simulink model "Model_complet"  (R2016a)
settings: Solver=VariableStepAuto  StartTime=0.0  StopTime=0.3  RelTol=1e-3
values from neighbouring files (symbols this model uses):
  Kid_ = 1*a1^2/e1    (= 5500.9287619)    [Data.m]
  Kiq_ = 1*b2^2/e2    (= 3122.67350797)    [Data.m]
  Pd_ = -1*a1/e1    (= 12.8976)    [Data.m]
  Pq_ = -1*b2/e2    (= 11.452173913)    [Data.m]
settings Model: Creator=NAD  LastModifiedBy=NAD

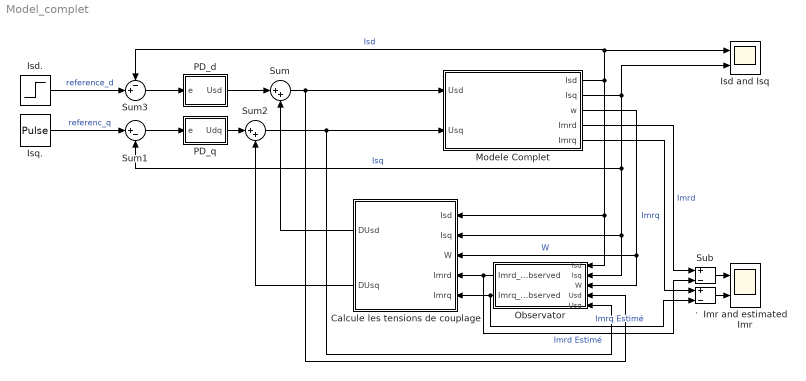
== system Model_complet ==
  . : Sum  Inputs=+-
  Calcule les tensions de couplage : MATLAB Function  TreatAsAtomicUnit=on
  Imr and estimated Imr : Scope  NumInputPorts=2
  Isd and Isq : Scope  NumInputPorts=2
  Isd. : Step  Time=0  After=10  SampleTime=0
  Isq. : DiscretePulseGenerator  PulseType=Time based  Amplitude=10  Period=0.2  PulseWidth=50
  Modele Complet : Subsystem
  Observator : Subsystem
  PD_d : Subsystem
  PD_q : Subsystem
  Sub : Sum  Inputs=+-
  Sum : Sum  Inputs=|++
  Sum1 : Sum  Inputs=|+-
  Sum2 : Sum  Inputs=|++
  Sum3 : Sum  Inputs=-+|
  wires:
  Modele Complet/1(Isd) -> Calcule les tensions de couplage/1(Isd), Observator/1(Isd), Sum3/1, Isd and Isq/1  "Isd"
  Modele Complet/3(w) -> Calcule les tensions de couplage/3(W), Observator/3(W)  "W"
  Sum3/1 -> PD_d/1(e)
  Sum1/1 -> PD_q/1(e)
  PD_d/1(Usd) -> Sum/1
  Sum/1 -> Observator/4(Usd), Modele Complet/1(Usd)
  Sum2/1 -> Observator/5(Usq), Modele Complet/2(Usq)
  PD_q/1(Udq) -> Sum2/1
  Calcule les tensions de couplage/1(DUsd) -> Sum/2
  Calcule les tensions de couplage/2(DUsq) -> Sum2/2
  Observator/1(Imrd_Observed) -> Sub/2, Calcule les tensions de couplage/4(Imrd)  "Imrd Estimé"
  Observator/2(Imrq_Observed) -> ./2, Calcule les tensions de couplage/5(Imrq)  "Imrq Estimé"
  Sub/1 -> Imr and estimated Imr/1
  Modele Complet/4(Imrd) -> Sub/1  "Imrd"
  Modele Complet/5(Imrq) -> ./1  "Imrq"
  ./1 -> Imr and estimated Imr/2
  Modele Complet/2(Isq) -> Sum1/2, Calcule les tensions de couplage/2(Isq), Observator/2(Isq), Isd and Isq/2  "Isq"
  Isq./1 -> Sum1/1  "referenc_q"
  Isd./1 -> Sum3/2  "reference_d"

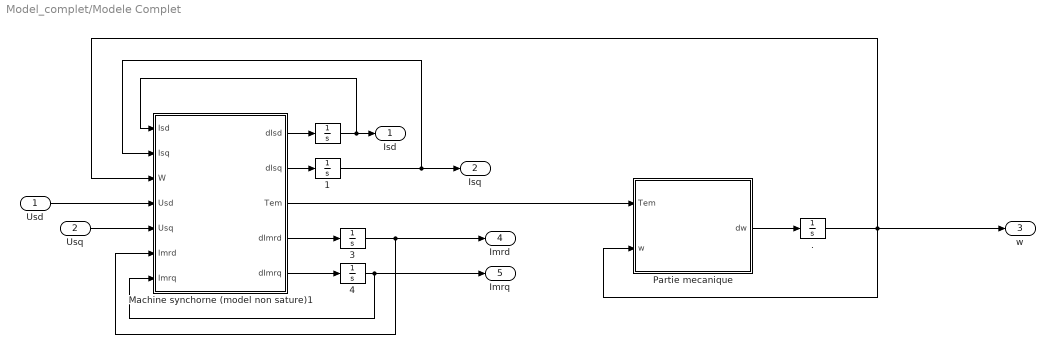
== system Model_complet/Modele Complet ==
  Usd : Inport
  Usq : Inport  Port=2
  " " : Integrator
  " ." : Integrator
  " 1" : Integrator
  " 3" : Integrator  InitialCondition=1
  " 4" : Integrator  InitialCondition=1
  Machine synchorne (model non sature)1 : MATLAB Function  TreatAsAtomicUnit=on
  Partie mecanique : MATLAB Function  TreatAsAtomicUnit=on
  Isd : Outport
  Isq : Outport  Port=2
  w : Outport  Port=3
  Imrd : Outport  Port=4
  Imrq : Outport  Port=5
  wires:
  Machine synchorne (model non sature)1/1(dIsd) -> " "/1
  " "/1 -> Isd/1, Machine synchorne (model non sature)1/1(Isd)
  " ."/1 -> w/1, Partie mecanique/2(w), Machine synchorne (model non sature)1/3(W)
  Partie mecanique/1(dw) -> " ."/1
  Machine synchorne (model non sature)1/3(Tem) -> Partie mecanique/1(Tem)
  Machine synchorne (model non sature)1/2(dIsq) -> " 1"/1
  " 1"/1 -> Machine synchorne (model non sature)1/2(Isq), Isq/1
  Usd/1 -> Machine synchorne (model non sature)1/4(Usd)
  Usq/1 -> Machine synchorne (model non sature)1/5(Usq)
  Machine synchorne (model non sature)1/4(dImrd) -> " 3"/1
  Machine synchorne (model non sature)1/5(dImrq) -> " 4"/1
  " 4"/1 -> Machine synchorne (model non sature)1/7(Imrq), Imrq/1
  " 3"/1 -> Imrd/1, Machine synchorne (model non sature)1/6(Imrd)

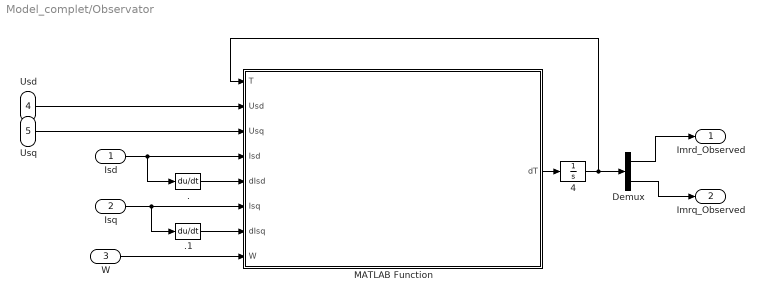
== system Model_complet/Observator ==
  Isd : Inport
  Isq : Inport  Port=2
  W : Inport  Port=3
  Usd : Inport  Port=4
  Usq : Inport  Port=5
  " 4" : Integrator  InitialCondition=0.01*[1;1]
  . : Derivative
  .1 : Derivative
  Demux : Demux  Outputs=2
  MATLAB Function : MATLAB Function  TreatAsAtomicUnit=on
  Imrd_Observed : Outport
  Imrq_Observed : Outport  Port=2
  wires:
  W/1 -> MATLAB Function/8(W)
  .1/1 -> MATLAB Function/7(dIsq)
  MATLAB Function/1(dT) -> " 4"/1
  " 4"/1 -> Demux/1, MATLAB Function/1(T)
  ./1 -> MATLAB Function/5(dIsd)
  Demux/1 -> Imrd_Observed/1
  Isq/1 -> .1/1, MATLAB Function/6(Isq)
  Isd/1 -> MATLAB Function/4(Isd), ./1
  Usd/1 -> MATLAB Function/2(Usd)
  Demux/2 -> Imrq_Observed/1
  Usq/1 -> MATLAB Function/3(Usq)

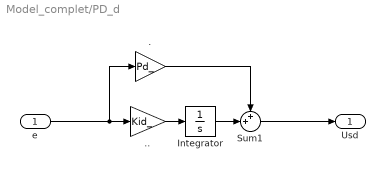
== system Model_complet/PD_d ==
  e : Inport
  ". " : Gain  Gain=Pd_
  .. : Gain  Gain=Kid_
  Integrator : Integrator
  Sum1 : Sum  Inputs=++|
  Usd : Outport
  wires:
  ../1 -> Integrator/1
  Integrator/1 -> Sum1/2
  ". "/1 -> Sum1/1
  e/1 -> ". "/1, ../1
  Sum1/1 -> Usd/1

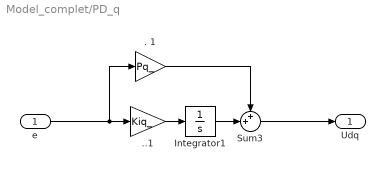
== system Model_complet/PD_q ==
  e : Inport
  . 1 : Gain  Gain=Pq_
  ..1 : Gain  Gain=Kiq_
  Integrator1 : Integrator
  Sum3 : Sum  Inputs=++|
  Udq : Outport
  wires:
  ..1/1 -> Integrator1/1
  e/1 -> ..1/1, . 1/1
  . 1/1 -> Sum3/1
  Integrator1/1 -> Sum3/2
  Sum3/1 -> Udq/1

== matlab function Model_complet/Modele Complet/Partie mecanique ==
  data: Tem input; w input; dw output
function dw  = fct(Tem,w)
%% Les parametres:
J = 0.05;
f = 0.002 ;

dw= -f/J*w + Tem/J;

== matlab function Model_complet/Modele Complet/Machine synchorne (model non sature)1 ==
  data: Isd input; Isq input; W input; Usd input; Usq input; dIsd output; dIsq output; Tem output; Imrd input; Imrq input; dImrd output; dImrq output
function [dIsd,dIsq,Tem,dImrd,dImrq] = fct(Isd,Isq,W,Usd,Usq,Imrd,Imrq)
%% Les parametres:
Rs=7.8;
Ld = 0.54 ;
wd=0.056;
Trd =0.1;
Lq=0.21;
wq=0.2;
Trq=0.046;

% Paramatres supposés :
p = 3; 
% la vitesse angulaire electrique:
we=p*W;
% le coeficient de transformation du champ magentique Imr d'une machine a poles saillants vers un chemp magnetisant magnetisant equivalent Imr_ d'une magine a pole sille
k=sqrt(Lq*(1-wq)/Ld/(1-wd));
% Le champs magnetisant equivalent:
Imr_ = sqrt(Imrd^2+Imrq^2*k^2);
% le coefficient de saturation Ks(Imr_) = N/D
a = -1.376 ; c =-0.0247 ; e= -1.381 ; g=-0.080;
b= 0.586 ; d= 0.005 ; f =0.619 ; h =0.033;
N = 1 + a*Imr_ + b*Imr_^2 + c*Imr_^3 + d*Imr_^4;
D = 1 + e*Imr_ + f*Imr_^2 + g*Imr_^3 + h*Imr_^4;
Ks = N/D;
% le coefficient de saturation dynamique Ksd(Imr_) = dKs/dImr_ 
dN = a + 2*b*Imr_ + 3*c*Imr_^2 + 4*d*Imr_^3;
dD = e + 2*f*Imr_ + 3*g*Imr_^2 + 4*h*Imr_^3;
Ksd = (dN*D-dD*N)/D^2;
% Ks= 1; Ksd =0.005;
% autre coefficients d'induction:
Ldd = Ld*(1-wd)*(Ks+Ksd*Imrd^2/Imr_);
Lqq = Lq*(1-wq)*(Ks+k^2*Ksd*Imrq^2/Imr_);
Mdq = Lq*(1-wq)*Ksd*Imrd*Imrq/Imr_;


%% le systeme 
% Les parametres de la matrce:
a1 = -(Rs/wd/Ld+(1-wd)/wd/Trd);b1= we*wq*Lq/wd/Ld; c1=(1-wd)/wd/Trd ;d1= Ks*we*Lq*(1-wq)/wd/Ld ; e1=1/(wd*Ld) ;
a2 =- we*wd*Ld/wq/Lq ;b2=-(Rs/wq/Lq+(1-wq)/wq/Trq) ; c2=- Ks*we*Ld*(1-wd)/wq/Lq ;d2= (1-wq)/wq/Trq; e2=1/(wq*Lq) ;
a3 = 1/(Ks*(Ks+Ksd*Imr_))*(Lqq/Trd/Lq/(1-wq)) ;b3= -1/(Ks*(Ks+Ksd*Imr_))*k^2*Mdq/Trq/Lq/(1-wq) ; c3= -a3; d3= -b3 ; 
a4 = -1/(Ks*(Ks+Ksd*Imr_))*Mdq/Trd/Lq/(1-wq);b4= 1/(Ks*(Ks+Ksd*Imr_))*(Ldd/Trq/Ld/(1-wd)); c4=-a4 ;d4=-b4 ; 

I=[Isd;Isq;Imrd;Imrq]; U = [Usd;Usq]; 
A= [a1 b1 c1 d1
    a2 b2 c2 d2
    a3 b3 c3 d3
    a4 b4 c4 d4];
B= [e1 0
    0 e2
    0 0
    0 0];
dI = A*I+B*U;
dIsd = dI(1);
dIsq = dI(2);
dImrd = dI(3);
dImrq = dI(4);

Tem = p*(Ld-Lq)*Isd*Isq;

% % les equations de courants statoriques:
% dIsd = -(Rs/wd/Ld+(1-wd)/wd/Trd)*Isd + we*wq*Lq/wd/Ld*Isq+(1-wd)/wd/Trd*Imrd + Ks*we*Lq*(1-wq)/wd/Ld*Imrq + 1/(wd*Ld)*Usd;
% dIsq = -(Rs/wq/Lq+(1-wq)/wq/Trq)*Isq - we*wd*Ld/wq/Lq*Isd+(1-wq)/wq/Trq*Imrq - Ks*we*Ld*(1-wd)/wq/Lq*Imrd + 1/(wq*Lq)*Usq;
% 
% % le courants de magnetisation:
% dImrd = 1/(Ks*(Ks+Ksd*Imr_))*(Lqq/Trd/Lq/(1-wq)*(Isd-Imrd)+k^2*Mdq/Trq/Lq/(1-wq)*(Imrq-Isq));
% dImrq = 1/(Ks*(Ks+Ksd*Imr_))*(Ldd/Trq/Ld/(1-wd)*(Isq-Imrq)+ Mdq/Trd/Lq/(1-wq)*(Imrd-Isd));
% 

% 
% 
% Imrd= Isd + Lrd/Md*ird;
% Imrq = Isq + Lrq/Md*irq;

== matlab function Model_complet/Observator/MATLAB Function ==
  data: T input; dT output; Usd input; Usq input; Isd input; dIsd input; Isq input; dIsq input; W input
    function dT = fct(T,Usd,Usq,Isd,dIsd,Isq,dIsq,W)
%% Les parametres:
Rs=7.8;
Ld = 0.54 ;
wd=0.056;
Trd =0.1;
Lq=0.21;
wq=0.2;
Trq=0.046;

% Paramatres supposés :
p = 3; 
% la vitesse angulaire electrique:
we=p*W;
% le coeficient de transformation du champ magentique Imr d'une machine a poles saillants vers un chemp magnetisant magnetisant equivalent Imr_ d'une magine a pole sille
k=sqrt(Lq*(1-wq)/Ld/(1-wd));
% Le champs magnetisant equivalent:
Imrd = T(1); Imrq=T(2);
Imr_ = sqrt(Imrd^2+Imrq^2*k^2);
% le coefficient de saturation Ks(Imr_) = N/D
a = -1.376 ; c =-0.0247 ; e= -1.381 ; g=-0.080;
b= 0.586 ; d= 0.005 ; f =0.619 ; h =0.033;
N = 1 + a*Imr_ + b*Imr_^2 + c*Imr_^3 + d*Imr_^4;
D = 1 + e*Imr_ + f*Imr_^2 + g*Imr_^3 + h*Imr_^4;
Ks = N/D;
% le coefficient de saturation dynamique Ksd(Imr_) = dKs/dImr_ 
dN = a + 2*b*Imr_ + 3*c*Imr_^2 + 4*d*Imr_^3;
dD = e + 2*f*Imr_ + 3*g*Imr_^2 + 4*h*Imr_^3;
Ksd = (dN*D-dD*N)/D^2;
% Ks= 1; Ksd =0.005;
% autre coefficients d'induction:
Ldd = Ld*(1-wd)*(Ks+Ksd*Imrd^2/Imr_);
Lqq = Lq*(1-wq)*(Ks+k^2*Ksd*Imrq^2/Imr_);
Mdq = Lq*(1-wq)*Ksd*Imrd*Imrq/Imr_;


%% le systeme 
% Les parametres de la matrce:
a1 = -(Rs/wd/Ld+(1-wd)/wd/Trd);b1= we*wq*Lq/wd/Ld; c1=(1-wd)/wd/Trd ;d1= Ks*we*Lq*(1-wq)/wd/Ld ; e1=1/(wd*Ld) ;
a2 =- we*wd*Ld/wq/Lq ;b2=-(Rs/wq/Lq+(1-wq)/wq/Trq) ; c2=- Ks*we*Ld*(1-wd)/wq/Lq ;d2= (1-wq)/wq/Trq; e2=1/(wq*Lq) ;
a3 = 1/(Ks*(Ks+Ksd*Imr_))*(Lqq/Trd/Lq/(1-wq)) ;b3= -1/(Ks*(Ks+Ksd*Imr_))*k^2*Mdq/Trq/Lq/(1-wq) ; c3= -a3; d3= -b3 ; 
a4 = -1/(Ks*(Ks+Ksd*Imr_))*Mdq/Trd/Lq/(1-wq);b4= 1/(Ks*(Ks+Ksd*Imr_))*(Ldd/Trq/Ld/(1-wd)); c4=-a4 ;d4=-b4 ; 


%%
Is = [Isd;Isq];
dIs = [dIsd;dIsq];
Us = [Usd;Usq];

Um = [a3 b3; a4 b4]*Is;
Ym = [c1 d1; c2 d2]\(dIs-[a1 b1; a2 b2]*Is-[e1 0 ;0 e2]*Us);
Am = [c3 d3; c4 d4];

l = 50;
Km = Am + [l 0; 0 l];
dT = -[l 0; 0 l]*T + Um + Km*Ym;

== matlab function Model_complet/Calcule les tensions de couplage ==
  data: Isd input; DUsd output; Isq input; W input; Imrd input; Imrq input; DUsq output
function [DUsd,DUsq] = fct(Isd,Isq,W,Imrd,Imrq)
%% Les parametres:
Rs=7.8;
Ld = 0.54 ;
wd=0.056;
Trd =0.1;
Lq=0.21;
wq=0.2;
Trq=0.046;

% Paramatres supposés :
p = 3; 
% la vitesse angulaire electrique:
we=p*W;
% le coeficient de transformation du champ magentique Imr d'une machine a poles saillants vers un chemp magnetisant magnetisant equivalent Imr_ d'une magine a pole sille
k=sqrt(Lq*(1-wq)/Ld/(1-wd));
% Le champs magnetisant equivalent:
Imr_ = sqrt(Imrd^2+Imrq^2*k^2);
% le coefficient de saturation Ks(Imr_) = N/D
a = -1.376 ; c =-0.0247 ; e= -1.381 ; g=-0.080;
b= 0.586 ; d= 0.005 ; f =0.619 ; h =0.033;
N = 1 + a*Imr_ + b*Imr_^2 + c*Imr_^3 + d*Imr_^4;
D = 1 + e*Imr_ + f*Imr_^2 + g*Imr_^3 + h*Imr_^4;
Ks = N/D;

%% le systeme 
% Les parametres de la matrce:
b1= we*wq*Lq/wd/Ld; c1=(1-wd)/wd/Trd ;d1= Ks*we*Lq*(1-wq)/wd/Ld ; e1=1/(wd*Ld) ;
a2 =- we*wd*Ld/wq/Lq ; c2=- Ks*we*Ld*(1-wd)/wq/Lq ;d2= (1-wq)/wq/Trq; e2=1/(wq*Lq) ;

% les equations de courants statoriques:
DUsd = -(b1*Isq + c1*Imrd + d1*Imrq)/e1;
DUsq = -(a2*Isd + c2*Imrd + d2*Imrq )/e2;
